simulink model "forward_feedback_control"  (R2020b)
settings: Solver=VariableStepAuto  StartTime=0.0  StopTime=10.0  RelTol=1e-3
values from neighbouring files (symbols this model uses):
  Ki = block.DialogPrm(2).Data(:)    [general_task_controller.m]    (also in task_controller.m = block.DialogPrm(3).Data(:))
  Kp = block.DialogPrm(1).Data(:)    [general_task_controller.m]    (also in task_controller.m = block.DialogPrm(2).Data(:))
settings Model: Creator=a302  LastModifiedBy=a302

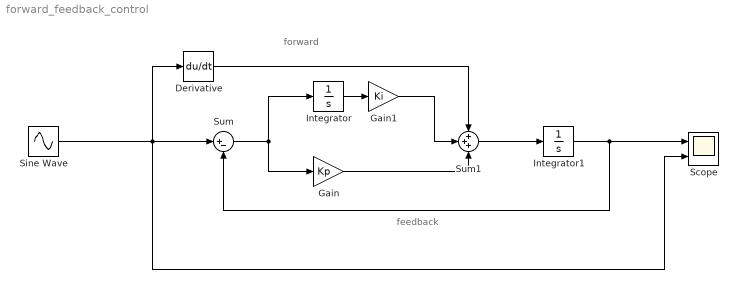
== system forward_feedback_control ==
  note: forward
  note: feedback
  Derivative : Derivative
  Gain : Gain  Gain=Kp
  Gain1 : Gain  Gain=Ki
  Integrator : Integrator
  Integrator1 : Integrator
  Scope : Scope  NumInputPorts=2
  Sine Wave : Sin  Frequency=5  SampleTime=0
  Sum : Sum  Inputs=|+-
  Sum1 : Sum  Inputs=+++
  wires:
  Sine Wave/1 -> Derivative/1, Sum/1, Scope/2
  Sum/1 -> Gain/1, Integrator/1
  Integrator/1 -> Gain1/1
  Gain/1 -> Sum1/3
  Sum1/1 -> Integrator1/1
  Gain1/1 -> Sum1/2
  Integrator1/1 -> Sum/2, Scope/1
  Derivative/1 -> Sum1/1
